simulink model "sistema_transmisor"  (R2024b)
settings: Solver=VariableStepAuto  StartTime=0.0  StopTime=0.05  RelTol=1e-3
undefined symbols (not defined in the file or in its folder): Ts
settings Model: Creator=RomaW11  LastModifiedBy=RomaW11

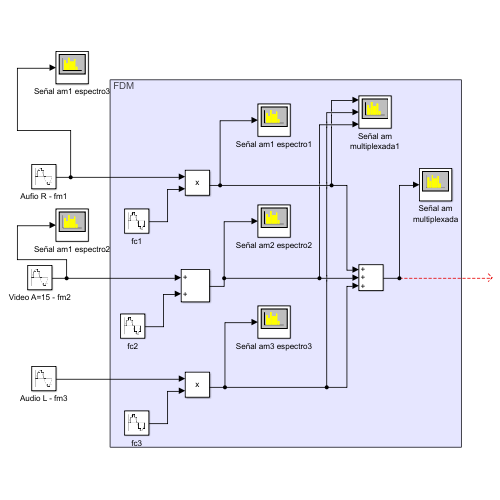
[thumbnail: Simulink's stored preview of the top-level diagram]
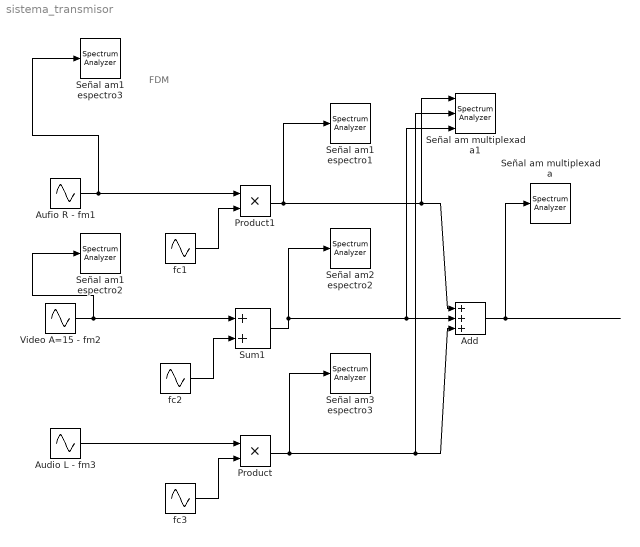
== system sistema_transmisor ==
  note: FDM
  Add : Sum  Inputs=+++
  Audio L - fm3 : Sin  Frequency=4800*2*pi  Phase=pi/2  SampleTime=Ts*0.5
  Aufio R - fm1 : Sin  Frequency=4500*2*pi  Phase=pi/2  SampleTime=Ts*0.5
  Product : Product
  Product1 : Product
  Señal am multiplexada : SpectrumAnalyzer  WindowPosition=[2.000000,50.000000,958.000000,1000.000000,]  Visible=on  ScopeFrameLocation=window  SampleRate=44.1e3  StartFrequency=20  StopFrequency=20e3  YLimits=[-251.58429751291825,58.34044322483905]  ShowLegend=on  SelectedToolstripTab=spectrumAnalyzerToolstrip.spectrumTab
      settings: OpenAtSimulationStart=off
  Señal am multiplexada1 : SpectrumAnalyzer  NumInputPorts=3  WindowPosition=[2.000000,50.000000,958.000000,1000.000000,]  Visible=on  ScopeFrameLocation=window  SampleRate=44.1e3  StartFrequency=20  StopFrequency=20e3  YLimits=[-268.62627739,56.49114064]  ShowLegend=on  SelectedToolstripTab=spectrumAnalyzerToolstrip.spectrumTab
      settings: OpenAtSimulationStart=off
  Señal am1 espectro1 : SpectrumAnalyzer  WindowPosition=[0.000000,12.000000,1920.000000,1057.000000,]  ScopeFrameLocation=window  SampleRate=44.1e3  StartFrequency=20  StopFrequency=20e3  YLimits=[-253.80039263,49.03867723]  ShowLegend=on  SelectedToolstripTab=spectrumAnalyzerToolstrip.spectrumTab
      settings: OpenAtSimulationStart=off
  Señal am1 espectro2 : SpectrumAnalyzer  WindowPosition=[2.000000,50.000000,958.000000,1000.000000,]  ScopeFrameLocation=window  SampleRate=44.1e3  StartFrequency=20  StopFrequency=20e3  YLimits=[-273.70235499,60.2034469]  ShowLegend=on  SelectedToolstripTab=spectrumAnalyzerToolstrip.channelMeasurementsTab
      settings: OpenAtSimulationStart=off
  Señal am1 espectro3 : SpectrumAnalyzer  WindowPosition=[10.000000,50.000000,1902.000000,1000.000000,]  ScopeFrameLocation=window  SampleRate=44.1e3  FrequencySpan=Span and center frequency  StartFrequency=20  StopFrequency=20e3  YLimits=[-152.46439105808838,229.56958198431204]  ShowLegend=on  SelectedToolstripTab=spectrumAnalyzerToolstrip.channelMeasurementsTab
      settings: OpenAtSimulationStart=off
  Señal am2 espectro2 : SpectrumAnalyzer  WindowPosition=[0.000000,12.000000,1920.000000,1057.000000,]  ScopeFrameLocation=window  SampleRate=44.1e3  StartFrequency=20  StopFrequency=20e3  YLimits=[-0.01158904,0.10430133]  ShowLegend=on  SelectedToolstripTab=spectrumAnalyzerToolstrip.spectrumTab
      settings: OpenAtSimulationStart=off
  Señal am3 espectro3 : SpectrumAnalyzer  WindowPosition=[0.000000,12.000000,1920.000000,1057.000000,]  ScopeFrameLocation=window  SampleRate=44.1e3  StartFrequency=20  StopFrequency=20e3  YLimits=[-0.00875564,0.07880078]  ShowLegend=on  SelectedToolstripTab=spectrumAnalyzerToolstrip.spectrumTab
      settings: OpenAtSimulationStart=off
  Sum1 : Sum
  Video A=15 - fm2 : Sin  Frequency=2*pi*3e6  Phase=pi/2  SampleTime=Ts*0.5
  fc1 : Sin  Frequency=2*pi*5.375e6  Phase=pi/2  SampleTime=Ts*0.5  VectorParams1D=off
  fc2 : Sin  Frequency=2*pi*1e6  Phase=pi/2  SampleTime=Ts*0.5
  fc3 : Sin  Frequency=2*pi*5.875e6  Phase=pi/2  SampleTime=Ts*0.5
  wires:
  Product/1 -> Señal am3 espectro3/1, Señal am multiplexada1/2, Add/3
  fc2/1 -> Sum1/2
  Aufio R - fm1/1 -> Señal am1 espectro3/1, Product1/1
  Audio L - fm3/1 -> Product/1
  Sum1/1 -> Señal am2 espectro2/1, Señal am multiplexada1/3, Add/2
  Product1/1 -> Señal am multiplexada1/1, Add/1, Señal am1 espectro1/1
  fc1/1 -> Product1/2
  fc3/1 -> Product/2
  Video A=15 - fm2/1 -> Señal am1 espectro2/1, Sum1/1
  Add/1 -> Señal am multiplexada/1
